simulink model "control_3quads_attached_outerloop"  (R2019a)
settings: Solver=FixedStepAuto  StartTime=0.0  StopTime=120  FixedStep=0.025  RelTol=1e-3  EnableMultiTasking=on
InitFcn:
  | global clientID;
  | clientID=-1;
values from neighbouring files (symbols this model uses):
  X = reshape(X, size(A_t))    [RiccatiCov.m]
undefined symbols (not defined in the file or in its folder): sigbuilder_block, Y, Z
libraries: robotlib x10, dspindex x3, simulink_extras x1
settings Model: Creator=Kleber Cabral  LastModifiedBy=Kleber Cabral
settings DataIOCC: SaveFormat=Array  ReturnWorkspaceOutputs=off
settings OptimizationCC: LifeSpan=inf
settings DebuggingCC: SolverPrmCheckMsg=warning  SFUnexpectedBacktrackingDiag=warning  SFNoUnconditionalDefaultTransitionDiag=warning  ArithmeticOperatorsInVariantConditions=warning
settings HardwareCC: ProdBitPerPointer=32  ProdBitPerSizeT=32  ProdBitPerPtrDiffT=32  ProdLargestAtomicFloat=None  ProdIntDivRoundTo=Undefined  ProdEndianess=Unspecified  ProdWordSize=32  ProdHWDeviceType=32-bit Generic
settings ModelReferenceCC: PropagateSignalLabelsOutOfModel=off
settings SFSimCC: SimUseLocalCustomCode=off
settings RTWCC: RTWUseLocalCustomCode=off
settings CodeAppCC: StateflowObjectComments=on
settings GRTTargetCC: TargetLangStandard=C89/C90 (ANSI)  GeneratePreprocessorConditionals=Disable all
settings ConfigComp: CovMetricSettings=dw  CovHtmlReporting=on  CovSaveCumulativeToWorkspaceVar=on  CovSaveSingleToWorkspaceVar=on  CovExternalEMLEnable=off  CovSFcnEnable=off

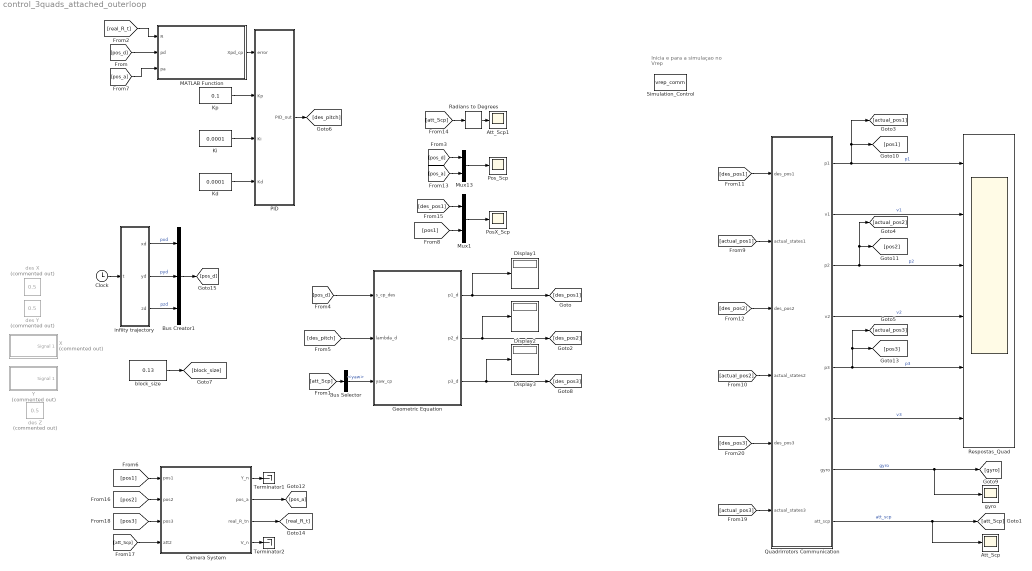
== system control_3quads_attached_outerloop ==
  note: Inicia e para a simulaçao no Vrep
  Att_Scp : Scope
  Att_Scp1 : Scope
  Bus Creator1 : BusCreator  Inputs=3
  Bus Selector : BusSelector  OutputSignals=yaw
  Camera System : Subsystem
  Clock : Clock
  Display1 : Display
      settings: Decimation=3
  Display2 : Display
      settings: Decimation=3
  Display3 : Display
      settings: Decimation=3
  Geometric Equation : MATLAB Function  TreatAsAtomicUnit=on
  Kd : Constant  Value=0.0001
  Ki : Constant  Value=0.0001
  Kp : Constant  Value=0.1
  MATLAB Function : MATLAB Function  TreatAsAtomicUnit=on
  Mux1 : Mux  Inputs=2
  Mux13 : Mux  Inputs=2
  PID : Subsystem
  PosX_Scp : Scope
  Pos_Scp : Scope
  Quadrirrotors Communication : Subsystem
  Radians to Degrees : simulink_extras/Transformations/Radians to Degrees
  Respostas_Quad : Scope  NumInputPorts=6
  Simulation_Control : S-Function  FunctionName=vrep_comm  SFunctionDeploymentMode=off  EnableBusSupport=off
  Terminator1 : Terminator
  Terminator2 : Terminator
  X : Subsystem  Tag=STV Subsys  Commented=on  LoadFcn=sigbuilder_block('load');  StartFcn=sigbuilder_block('start');  StopFcn=sigbuilder_block('stop');  ClipboardFcn=sigbuilder_block('clipboard');  mask(Sigbuilder block){tuvar=[0:10]}
      mask help: Simulink:masks:SigbuilderBlock_MD
      mask init:
      | if ~strcmp(get_param(bdroot(gcbh),'SimulationStatus'),'stopped') tuvar = sigbuilder_block('maskInit'); end
      settings: CopyFcn=sigbuilder_block('copy');  DeleteFcn=sigbuilder_block('delete');  ModelCloseFcn=sigbuilder_block('modelClose');  PreSaveFcn=sigbuilder_block('preSave');  PauseFcn=sigbuilder_block('pause');  ContinueFcn=sigbuilder_block('continue');  NameChangeFcn=sigbuilder_block('namechange');  OpenFcn=sigbuilder_block('open',[46.5 0 1393.5 843 ]);  CloseFcn=sigbuilder_block('close');
      mask Display: plot(0, 0, 100, 100,[2, 2, 32, 32, 2], [68, 8, 8, 68, 68],[32, 2], [38, 38], [32, 19, 2],[53, 60, 44], [32, 17, 17, 2],[16, 16, 31, 31]);txt = getActiveGroup(gcbh);text(2, 100, txt,'verticalAlignment', 'top');
  Y : Subsystem  Tag=STV Subsys  Commented=on  LoadFcn=sigbuilder_block('load');  StartFcn=sigbuilder_block('start');  StopFcn=sigbuilder_block('stop');  ClipboardFcn=sigbuilder_block('clipboard');  mask(Sigbuilder block){tuvar=[0:10]}
      mask help: Simulink:masks:SigbuilderBlock_MD
      mask init:
      | if ~strcmp(get_param(bdroot(gcbh),'SimulationStatus'),'stopped') tuvar = sigbuilder_block('maskInit'); end
      settings: CopyFcn=sigbuilder_block('copy');  DeleteFcn=sigbuilder_block('delete');  ModelCloseFcn=sigbuilder_block('modelClose');  PreSaveFcn=sigbuilder_block('preSave');  PauseFcn=sigbuilder_block('pause');  ContinueFcn=sigbuilder_block('continue');  NameChangeFcn=sigbuilder_block('namechange');  OpenFcn=sigbuilder_block('open',[40.5 0 1393.5 802.5 ]);  CloseFcn=sigbuilder_block('close');
      mask Display: plot(0, 0, 100, 100,[2, 2, 32, 32, 2], [68, 8, 8, 68, 68],[32, 2], [38, 38], [32, 19, 2],[53, 60, 44], [32, 17, 17, 2],[16, 16, 31, 31]);txt = getActiveGroup(gcbh);text(2, 100, txt,'verticalAlignment', 'top');
  block_size : Constant  Value=0.13
  des X : Constant  Commented=on  Value=0.5
  des Y : Constant  Commented=on  Value=0.5
  des Z : Constant  Commented=on  Value=0.5
  gyro : Scope
  infiity trajectory : MATLAB Function  TreatAsAtomicUnit=on
  wires:
  Kp/1 -> PID/2(Kp)
  Ki/1 -> PID/3(Ki)
  Kd/1 -> PID/4(Kd)
  infiity trajectory/1(xd) -> Bus Creator1/1  "pxd"
  infiity trajectory/2(yd) -> Bus Creator1/2  "pyd"
  infiity trajectory/3(zd) -> Bus Creator1/3  "pzd"
  PID/1(PID_out) -> [des_pitch]
  block_size/1 -> [block_size]
  [des_pitch] -> Geometric Equation/2(lambda_d)
  [att_Scp] -> Bus Selector/1
  [actual_pos1] -> Quadrirrotors Communication/2(actual_states1)
  Quadrirrotors Communication/7(gyro) -> gyro/1, [gyro]  "gyro"
  Quadrirrotors Communication/4(v2) -> Respostas_Quad/4  "v2"
  [des_pos1] -> Quadrirrotors Communication/1(des_pos1)
  [des_pos3] -> Quadrirrotors Communication/5(des_pos3)
  Quadrirrotors Communication/2(v1) -> Respostas_Quad/2  "v1"
  Quadrirrotors Communication/1(p1) -> Respostas_Quad/1, [actual_pos1], [pos1]  "p1"
  [actual_pos3] -> Quadrirrotors Communication/6(actual_states3)
  [des_pos2] -> Quadrirrotors Communication/3(des_pos2)
  Quadrirrotors Communication/3(p2) -> Respostas_Quad/3, [actual_pos2], [pos2]  "p2"
  Quadrirrotors Communication/8(att_scp) -> Att_Scp/1, [att_Scp]  "att_scp"
  Quadrirrotors Communication/5(p3) -> Respostas_Quad/5, [actual_pos3], [pos3]  "p3"
  [actual_pos2] -> Quadrirrotors Communication/4(actual_states2)
  Quadrirrotors Communication/6(v3) -> Respostas_Quad/6  "v3"
  Geometric Equation/1(p1_d) -> Display1/1, [des_pos1]
  Bus Selector/1 -> Geometric Equation/3(yaw_cp)  "<yaw>"
  Geometric Equation/2(p2_d) -> Display2/1, [des_pos2]
  Geometric Equation/3(p3_d) -> Display3/1, [des_pos3]
  [att_Scp] -> Radians to Degrees/1
  Radians to Degrees/1 -> Att_Scp1/1
  [pos_d] -> Mux13/1
  Mux13/1 -> Pos_Scp/1
  [pos_a] -> Mux13/2
  [att_Scp] -> Camera System/4(att2)
  [pos2] -> Camera System/2(pos2)
  Camera System/3(real_R_tn) -> [real_R_t]
  [pos1] -> Camera System/1(pos1)
  [pos3] -> Camera System/3(pos3)
  Camera System/2(pos_a) -> [pos_a]
  Camera System/4(V_n) -> Terminator2/1
  Camera System/1(Y_n) -> Terminator1/1
  Bus Creator1/1 -> [pos_d]
  [pos_d] -> Geometric Equation/1(s_cp_des)
  [pos_d] -> MATLAB Function/2(pd)
  [real_R_t] -> MATLAB Function/1(R)
  MATLAB Function/1(Xpd_cp) -> PID/1(error)
  [pos_a] -> MATLAB Function/3(pa)
  Mux1/1 -> PosX_Scp/1
  [pos1] -> Mux1/2
  [des_pos1] -> Mux1/1
  Clock/1 -> infiity trajectory/1(t)

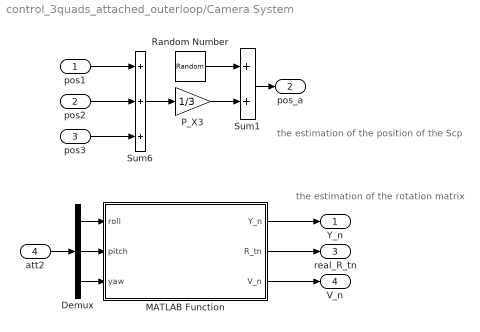
== system control_3quads_attached_outerloop/Camera System ==
  note: the estimation of the rotation matrix
  note: the estimation of the position of the Scp
  pos1 : Inport
  pos2 : Inport  Port=2
  pos3 : Inport  Port=3
  att2 : Inport  Port=4
  Demux : Demux  Outputs=3
  MATLAB Function : MATLAB Function  TreatAsAtomicUnit=on
  P_X3 : Gain  Gain=1/3
  Random Number : RandomNumber  Variance=0.03
  Sum1 : Sum
  Sum6 : Sum  Inputs=+++
  Y_n : Outport
  pos_a : Outport  Port=2
  real_R_tn : Outport  Port=3
  V_n : Outport  Port=4
  wires:
  pos1/1 -> Sum6/1
  pos2/1 -> Sum6/2
  Sum6/1 -> P_X3/1
  Sum1/1 -> pos_a/1
  att2/1 -> Demux/1
  Demux/3 -> MATLAB Function/3(yaw)
  Demux/2 -> MATLAB Function/2(pitch)
  Demux/1 -> MATLAB Function/1(roll)
  MATLAB Function/1(Y_n) -> Y_n/1
  MATLAB Function/2(R_tn) -> real_R_tn/1
  MATLAB Function/3(V_n) -> V_n/1
  pos3/1 -> Sum6/3
  P_X3/1 -> Sum1/2
  Random Number/1 -> Sum1/1

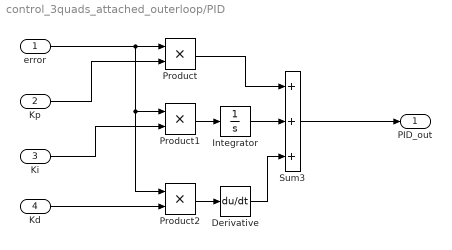
== system control_3quads_attached_outerloop/PID ==
  error : Inport
  Kp : Inport  Port=2
  Ki : Inport  Port=3
  Kd : Inport  Port=4
  Derivative : Derivative
  Integrator : Integrator
  Product : Product
  Product1 : Product
  Product2 : Product
  Sum3 : Sum  Inputs=+++
  PID_out : Outport
  wires:
  Kd/1 -> Product2/2
  Integrator/1 -> Sum3/2
  Product2/1 -> Derivative/1
  error/1 -> Product/1, Product2/1, Product1/1
  Product/1 -> Sum3/1
  Kp/1 -> Product/2
  Sum3/1 -> PID_out/1
  Ki/1 -> Product1/2
  Product1/1 -> Integrator/1
  Derivative/1 -> Sum3/3

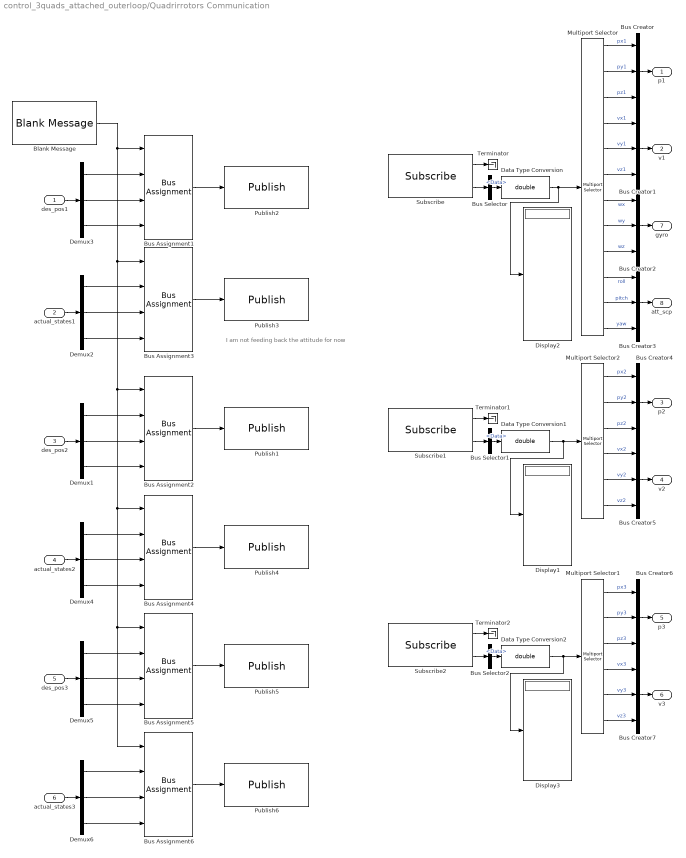
== system control_3quads_attached_outerloop/Quadrirrotors Communication ==
  note: I am not feeding back the attitude for now
  des_pos1 : Inport
  actual_states1 : Inport  Port=2
  des_pos2 : Inport  Port=3
  actual_states2 : Inport  Port=4
  des_pos3 : Inport  Port=5
  actual_states3 : Inport  Port=6
  Blank Message : robotlib/Blank Message  messageClass=Message  entityType=geometry_msgs/Vector3  messageType=geometry_msgs/Vector3  SampleTime=inf
      settings: SourceProductBaseCode=RO
  Bus Assignment{1..6} (6 alike) : BusAssignment  DialogController=Simulink.DDGSource_BusAssignment  AssignedSignals=X,Y,Z
  Bus Creator{,1..7} (8 alike) : BusCreator  Inputs=3
  Bus Selector : BusSelector  OutputSignals=Data
  Bus Selector1 : BusSelector  OutputSignals=Data
  Bus Selector2 : BusSelector  OutputSignals=Data
  Data Type Conversion : DataTypeConversion  OutDataTypeStr=double
  Data Type Conversion1 : DataTypeConversion  OutDataTypeStr=double
  Data Type Conversion2 : DataTypeConversion  OutDataTypeStr=double
  Demux{1..6} (6 alike) : Demux  Outputs=3
  Display1 : Display
      settings: Decimation=3
  Display2 : Display
      settings: Decimation=3
  Display3 : Display
      settings: Decimation=3
  Multiport Selector : dspindex/Multiport Selector  rowsOrCols=Rows  idxCellArray={1,2,3,4,5,6,7,8,9,10,11,12}  idxErrMode=Clip Index
  Multiport Selector1 : dspindex/Multiport Selector  rowsOrCols=Rows  idxCellArray={1,2,3,4,5,6}  idxErrMode=Clip Index
  Multiport Selector2 : dspindex/Multiport Selector  rowsOrCols=Rows  idxCellArray={1,2,3,4,5,6}  idxErrMode=Clip Index
  Publish1 : robotlib/Publish  topicSource=Select from ROS network  topic=/desired_waypoint_1  messageType=geometry_msgs/Vector3  messageQueueLength=105
      settings: SourceProductBaseCode=RO
  Publish2 : robotlib/Publish  topicSource=Select from ROS network  topic=/desired_waypoint_0  messageType=geometry_msgs/Vector3  messageQueueLength=105
      settings: SourceProductBaseCode=RO
  Publish3 : robotlib/Publish  topicSource=Select from ROS network  topic=/actual_states_0  messageType=geometry_msgs/Vector3  messageQueueLength=105
      settings: SourceProductBaseCode=RO
  Publish4 : robotlib/Publish  topicSource=Select from ROS network  topic=/actual_states_1  messageType=geometry_msgs/Vector3  messageQueueLength=105
      settings: SourceProductBaseCode=RO
  Publish5 : robotlib/Publish  topicSource=Select from ROS network  topic=/desired_waypoint_2  messageType=geometry_msgs/Vector3  messageQueueLength=105
      settings: SourceProductBaseCode=RO
  Publish6 : robotlib/Publish  topicSource=Select from ROS network  topic=/actual_states_2  messageType=geometry_msgs/Vector3  messageQueueLength=105
      settings: SourceProductBaseCode=RO
  Subscribe : robotlib/Subscribe  topicSource=Select from ROS network  topic=/quadrotor_states_0  messageType=std_msgs/Float32MultiArray  sampleTime=-1  messageQueueLength=51
      settings: SourceProductBaseCode=RO
  Subscribe1 : robotlib/Subscribe  topicSource=Select from ROS network  topic=/quadrotor_states_1  messageType=std_msgs/Float32MultiArray  sampleTime=-1  messageQueueLength=51
      settings: SourceProductBaseCode=RO
  Subscribe2 : robotlib/Subscribe  topicSource=Select from ROS network  topic=/quadrotor_states_2  messageType=std_msgs/Float32MultiArray  sampleTime=-1  messageQueueLength=51
      settings: SourceProductBaseCode=RO
  Terminator : Terminator
  Terminator1 : Terminator
  Terminator2 : Terminator
  p1 : Outport
  v1 : Outport  Port=2
  p2 : Outport  Port=3
  v2 : Outport  Port=4
  p3 : Outport  Port=5
  v3 : Outport  Port=6
  gyro : Outport  Port=7
  att_scp : Outport  Port=8
  wires:
  Subscribe/1 -> Terminator/1
  Subscribe/2 -> Bus Selector/1
  Data Type Conversion/1 -> Display2/1, Multiport Selector/1
  Bus Selector/1 -> Data Type Conversion/1  "<Data>"
  Bus Assignment1/1 -> Publish2/1
  Bus Assignment2/1 -> Publish1/1
  Subscribe1/1 -> Terminator1/1
  Subscribe1/2 -> Bus Selector1/1
  Data Type Conversion1/1 -> Display1/1, Multiport Selector2/1
  Bus Selector1/1 -> Data Type Conversion1/1  "<Data>"
  des_pos1/1 -> Demux3/1
  Demux3/1 -> Bus Assignment1/2
  Demux3/2 -> Bus Assignment1/3
  Demux3/3 -> Bus Assignment1/4
  des_pos2/1 -> Demux1/1
  Demux1/1 -> Bus Assignment2/2
  Demux1/2 -> Bus Assignment2/3
  Demux1/3 -> Bus Assignment2/4
  Demux2/3 -> Bus Assignment3/4
  Demux2/2 -> Bus Assignment3/3
  Demux2/1 -> Bus Assignment3/2
  actual_states1/1 -> Demux2/1
  Bus Assignment3/1 -> Publish3/1
  Demux4/3 -> Bus Assignment4/4
  Demux4/2 -> Bus Assignment4/3
  Demux4/1 -> Bus Assignment4/2
  actual_states2/1 -> Demux4/1
  Bus Assignment4/1 -> Publish4/1
  Bus Assignment6/1 -> Publish6/1
  actual_states3/1 -> Demux6/1
  Demux6/1 -> Bus Assignment6/2
  Demux6/2 -> Bus Assignment6/3
  Demux6/3 -> Bus Assignment6/4
  Demux5/3 -> Bus Assignment5/4
  Demux5/2 -> Bus Assignment5/3
  Demux5/1 -> Bus Assignment5/2
  des_pos3/1 -> Demux5/1
  Bus Assignment5/1 -> Publish5/1
  Blank Message/1 -> Bus Assignment3/1, Bus Assignment5/1, Bus Assignment6/1, Bus Assignment4/1, Bus Assignment2/1, Bus Assignment1/1
  Bus Selector2/1 -> Data Type Conversion2/1  "<Data>"
  Data Type Conversion2/1 -> Multiport Selector1/1, Display3/1
  Subscribe2/2 -> Bus Selector2/1
  Subscribe2/1 -> Terminator2/1
  Multiport Selector/3 -> Bus Creator/3  "pz1"
  Multiport Selector/2 -> Bus Creator/2  "py1"
  Bus Creator/1 -> p1/1
  Multiport Selector/6 -> Bus Creator1/3  "vz1"
  Multiport Selector/4 -> Bus Creator1/1  "vx1"
  Multiport Selector/5 -> Bus Creator1/2  "vy1"
  Bus Creator1/1 -> v1/1
  Multiport Selector2/2 -> Bus Creator4/2  "py2"
  Multiport Selector2/3 -> Bus Creator4/3  "pz2"
  Multiport Selector2/1 -> Bus Creator4/1  "px2"
  Bus Creator4/1 -> p2/1
  Multiport Selector2/4 -> Bus Creator5/1  "vx2"
  Multiport Selector2/5 -> Bus Creator5/2  "vy2"
  Multiport Selector2/6 -> Bus Creator5/3  "vz2"
  Bus Creator5/1 -> v2/1
  Bus Creator7/1 -> v3/1
  Multiport Selector1/6 -> Bus Creator7/3  "vz3"
  Multiport Selector1/5 -> Bus Creator7/2  "vy3"
  Multiport Selector1/4 -> Bus Creator7/1  "vx3"
  Bus Creator6/1 -> p3/1
  Multiport Selector1/1 -> Bus Creator6/1  "px3"
  Multiport Selector1/3 -> Bus Creator6/3  "pz3"
  Multiport Selector1/2 -> Bus Creator6/2  "py3"
  Multiport Selector/7 -> Bus Creator2/1  "wx"
  Multiport Selector/8 -> Bus Creator2/2  "wy"
  Multiport Selector/9 -> Bus Creator2/3  "wz"
  Bus Creator2/1 -> gyro/1
  Multiport Selector/10 -> Bus Creator3/1  "roll"
  Multiport Selector/11 -> Bus Creator3/2  "pitch"
  Multiport Selector/12 -> Bus Creator3/3  "yaw"
  Bus Creator3/1 -> att_scp/1
  Multiport Selector/1 -> Bus Creator/1  "px1"

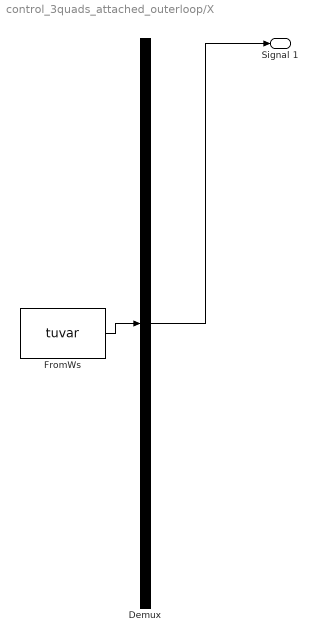
== system control_3quads_attached_outerloop/X ==
  Demux : Demux  Tag=STV Demux  Outputs=1
  FromWs : FromWorkspace  Tag=STV FromWs  VariableName=tuvar  SampleTime=0
      SigBuilderData=|
      | common.afterFinalStr = 'Extrapolate'
      | common.sampleTime = 0
      | dataSet.timeRange = [0 60]
      | dataSet.name = 'Group 1'
      | sbobj.Groups.Name = 'Group 1'
      | sbobj.Groups.Signals.Name = 'Signal 1'
      | sbobj.Groups.Signals.XData = [0 20 20.3 20.5 29.55 29.75 30 40 40.2 40.35 49.55 49.75 50 60]
      | sbobj.Groups.Signals.YData = [0 0 0.008 0.018 0.98 0.992 1 1 0.994 0.986 0.02 0.008 0 0]
      | sbobj.Groups.TimeRange = [0 60]
  Signal 1 : Outport  Tag=STV Outport
  wires:
  Demux/1 -> Signal 1/1
  FromWs/1 -> Demux/1

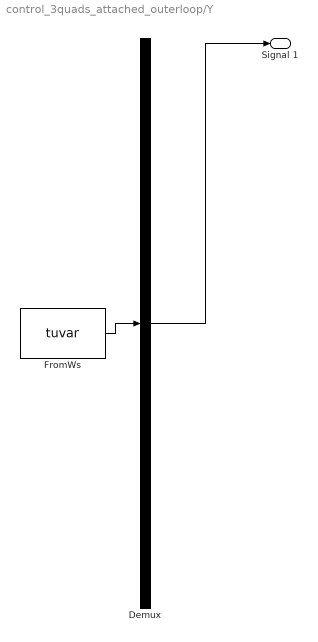
== system control_3quads_attached_outerloop/Y ==
  Demux : Demux  Tag=STV Demux  Outputs=1
  FromWs : FromWorkspace  Tag=STV FromWs  VariableName=tuvar  SampleTime=0
      SigBuilderData=|
      | common.afterFinalStr = 'Extrapolate'
      | common.sampleTime = 0
      | dataSet.timeRange = [0 60]
      | dataSet.name = 'Group 1'
      | sbobj.Groups.Name = 'Group 1'
      | sbobj.Groups.Signals.Name = 'Signal 1'
      | sbobj.Groups.Signals.XData = [0 10 10.3 10.5 19.55 19.75 20 40 40.2 40.35 49.55 49.75 50 60]
      | sbobj.Groups.Signals.YData = [0 0 0.008 0.018 0.98 0.99 1 1 0.994 0.986 0.02 0.008 0 0]
      | sbobj.Groups.TimeRange = [0 60]
  Signal 1 : Outport  Tag=STV Outport
  wires:
  FromWs/1 -> Demux/1
  Demux/1 -> Signal 1/1

== matlab function control_3quads_attached_outerloop/Camera System/MATLAB Function ==
  data: roll input; Y_n output; pitch input; yaw input; R_tn output; V_n output
function [Y_n,R_tn,V_n] = EulerAng2RotMat(roll, pitch, yaw)
% a=deg2rad(0);
% b=deg2rad(0);
% c=deg2rad(45);

a=roll;
b=pitch;
c=yaw;

sa=sin(a);ca=cos(a);
sb=sin(b);cb=cos(b);
sc=sin(c);cc=cos(c);
R_tn=[ cc*cb cc*sb*sa-sc*ca cc*sb*ca+sc*sa 
    sc*cb sc*sb*sa+cc*ca sc*sb*ca-cc*sa 
    -sb       cb*sa           cb*ca     ];

%noise of about 1 deg of rotation in each axis
a=deg2rad(randn*5);
b=deg2rad(randn*5);
c=deg2rad(randn*5);
sa=sin(a);ca=cos(a);
sb=sin(b);cb=cos(b);
sc=sin(c);cc=cos(c);
V_n=[ cc*cb cc*sb*sa-sc*ca cc*sb*ca+sc*sa 
    sc*cb sc*sb*sa+cc*ca sc*sb*ca-cc*sa 
    -sb       cb*sa           cb*ca     ];

Y_n = R_tn * V_n;

%R = R *(eye(3)+0.001*randn(3,3));
end

== matlab function control_3quads_attached_outerloop/Geometric Equation ==
  data: s_cp_des input; p1_d output; p2_d output; p3_d output; lambda_d input; yaw_cp input
function [p1_d,p2_d,p3_d] = fcn(s_cp_des,lambda_d,yaw_cp)
%#codegen

% s_cp_des=[u(1); u(2); u(3)];
% lambda_d=u(4);
% yaw_cp = u(5);

x1_cp=-0.13;
x2_cp=0;
x3_cp=0.13;

p1_d=s_cp_des + x1_cp*[cos(yaw_cp);sin(yaw_cp);-lambda_d];
p2_d=s_cp_des + x2_cp*[cos(yaw_cp);sin(yaw_cp);-lambda_d];
p3_d=s_cp_des + x3_cp*[cos(yaw_cp);sin(yaw_cp);-lambda_d];
%y=[eye(3);eye(3)]*[u(1);u(2);u(3)] + [-1;0;0;1;0;0]*(u(4)/2)+[0;0;1;0;0;-1]*u(5);

== matlab function control_3quads_attached_outerloop/MATLAB Function ==
  data: R input; Xpd_cp output; pd input; pa input
function Xpd_cp  = rotate2CPframe(R,pd,pa)
pd = [pd(1);pd(2);pd(3)];
pa = [pa(1);pa(2);pa(3)];
pd_cp=R*(pd-pa);

Xpd_cp=pd_cp(1);
end

== matlab function control_3quads_attached_outerloop/infiity trajectory ==
  data: t input; xd output; yd output; zd output
function [xd,yd,zd] = fcn(t)
%#codegen
t=t/10+deg2rad(90);
a=1;
xd=(a*cos(t))/(1+sin(t)^2);
yd=(a*sin(t)*cos(t))/(1+sin(t)^2);
zd=0.5;
